simulink model "vrepRotor"  (R2018a)
settings: Solver=FixedStepAuto  StartTime=0.0  StopTime=1.0  FixedStep=0.005  RelTol=1e-3
values from neighbouring files (symbols this model uses):
  clientID = block.InputPort(5).Data    [vrepConnection_Sfun.m]    (also in vrepQuadrotor.m = vrep.simxStart('127.0.0.1',19997,true,true,5000,5); vrepSlxInit.m = vrep.simxStart('127.0.0.1',19997,true,true,5000,5))
settings Model: Creator=dinies33  LastModifiedBy=dinies33

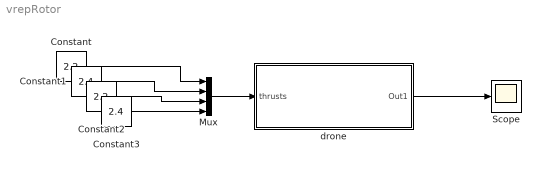
== system vrepRotor ==
  Constant : Constant  Value=2.2
  Constant1 : Constant  Value=2.4
  Constant2 : Constant  Value=2.2
  Constant3 : Constant  Value=2.4
  Mux : Mux
  Scope : Scope
  "drone " : Subsystem
  wires:
  Constant3/1 -> Mux/4
  Constant2/1 -> Mux/3
  Constant1/1 -> Mux/2
  Constant/1 -> Mux/1
  Mux/1 -> "drone "/1(thrusts)
  "drone "/1(Out1) -> Scope/1

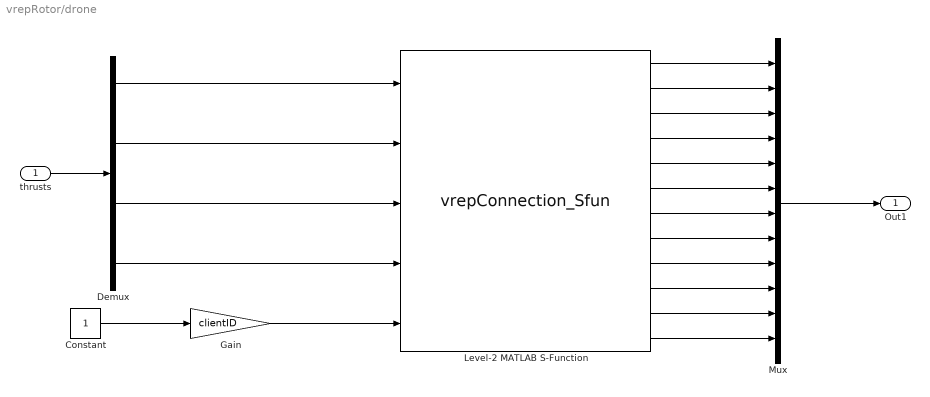
== system vrepRotor/drone  ==
  thrusts : Inport
  Constant : Constant
  Demux : Demux
  Gain : Gain  Gain=clientID
  Level-2 MATLAB S-Function : M-S-Function  FunctionName=vrepConnection_Sfun
  Mux : Mux  Inputs=12
  Out1 : Outport
  wires:
  thrusts/1 -> Demux/1
  Demux/1 -> Level-2 MATLAB S-Function/1
  Demux/2 -> Level-2 MATLAB S-Function/2
  Demux/3 -> Level-2 MATLAB S-Function/3
  Demux/4 -> Level-2 MATLAB S-Function/4
  Constant/1 -> Gain/1
  Gain/1 -> Level-2 MATLAB S-Function/5
  Level-2 MATLAB S-Function/8 -> Mux/8
  Level-2 MATLAB S-Function/7 -> Mux/7
  Level-2 MATLAB S-Function/6 -> Mux/6
  Level-2 MATLAB S-Function/5 -> Mux/5
  Level-2 MATLAB S-Function/4 -> Mux/4
  Level-2 MATLAB S-Function/3 -> Mux/3
  Level-2 MATLAB S-Function/2 -> Mux/2
  Level-2 MATLAB S-Function/1 -> Mux/1
  Level-2 MATLAB S-Function/12 -> Mux/12
  Level-2 MATLAB S-Function/11 -> Mux/11
  Level-2 MATLAB S-Function/9 -> Mux/9
  Level-2 MATLAB S-Function/10 -> Mux/10
  Mux/1 -> Out1/1
